simulink model "LQR_Kalman"  (R2024b)
settings: Solver=VariableStepAuto  StartTime=0.0  StopTime=tf  FixedStep=0.01  MaxStep=tf/1e4  RelTol=1e-4  AbsTol=1e-4
values from neighbouring files (symbols this model uses):
  A = [0 1; 0 0]    [Main_LQR_Kalman.m]    (also in dfdx.m = zeros(2))
  A_obs = A    [Main_LQR_Kalman.m]
  Bx = [0; Cx]    [Main_LQR_Kalman.m]
  Bx_obs = [Bx Kx_obs]    [Main_LQR_Kalman.m]
  By = [0; Cy]    [Main_LQR_Kalman.m]
  By_obs = [By Ky_obs]    [Main_LQR_Kalman.m]
  C = [1 0]    [Main_LQR_Kalman.m]
  C_obs = eye(2)    [Main_LQR_Kalman.m]
  D_obs = zeros(2)    [Main_LQR_Kalman.m]
  data_sys = [m r g J b lx ly]    [Main_LQR_Kalman.m]
  ICx_obs = [0 0]'    [Main_LQR_Kalman.m]
  ICy_obs = [0 0]'    [Main_LQR_Kalman.m]
  zx0 = [0.05,0]'    [Main_LQR_Kalman.m]
  zy0 = [0,0]'    [Main_LQR_Kalman.m]
settings Model: Creator=nicvi  LastModifiedBy=nicvi
settings SolverCC: AutoScaleAbsTol=off

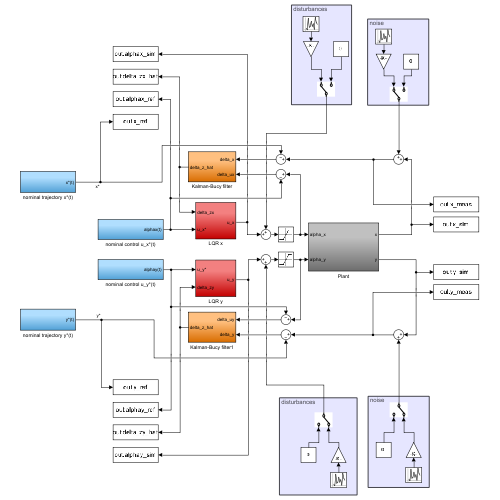
[thumbnail: Simulink's stored preview of the top-level diagram]
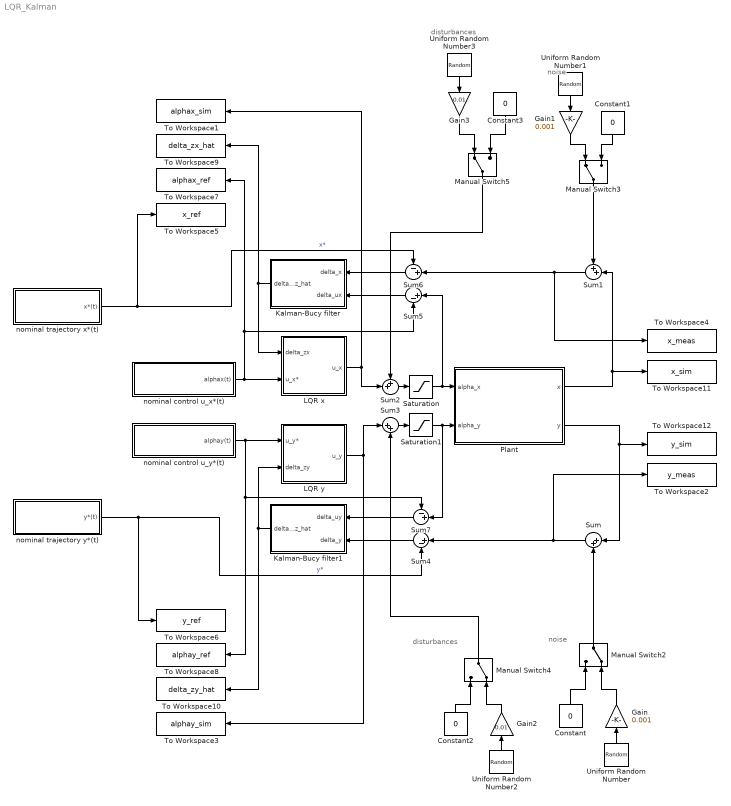
== system LQR_Kalman ==
  note: noise
  note: noise
  note: disturbances
  note: disturbances
  Constant{,1..3} (4 alike) : Constant  Value=0
  Gain : Gain  Gain=0.001
  Gain1 : Gain  Gain=0.001
  Gain2 : Gain  Gain=0.01
  Gain3 : Gain  Gain=0.01
  Kalman-Bucy filter : Subsystem
  Kalman-Bucy filter1 : Subsystem
  LQR x : Subsystem
  LQR y : Subsystem
  Manual Switch2 : ManualSwitch  CurrentSetting=0
  Manual Switch3 : ManualSwitch
  Manual Switch4 : ManualSwitch  CurrentSetting=0
  Manual Switch5 : ManualSwitch
  Plant : Subsystem
  Saturation : Saturate  UpperLimit=deg2rad(75)  LowerLimit=deg2rad(-75)
  Saturation1 : Saturate  UpperLimit=deg2rad(75)  LowerLimit=deg2rad(-75)
  Sum : Sum  Inputs=|++
  Sum1 : Sum  Inputs=++|
  Sum2 : Sum  Inputs=++|
  Sum3 : Sum  Inputs=|++
  Sum4 : Sum  Inputs=|+-
  Sum5 : Sum  Inputs=|+-
  Sum6 : Sum  Inputs=-+|
  Sum7 : Sum  Inputs=-+|
  To Workspace1 : ToWorkspace  VariableName=alphax_sim  SampleTime=-1
      settings: Save2DSignal=2-D array (concatenate along first dimension)
  To Workspace10 : ToWorkspace  VariableName=delta_zy_hat  SampleTime=-1
      settings: Save2DSignal=2-D array (concatenate along first dimension)
  To Workspace11 : ToWorkspace  VariableName=x_sim  SampleTime=-1
      settings: Save2DSignal=2-D array (concatenate along first dimension)
  To Workspace12 : ToWorkspace  VariableName=y_sim  SampleTime=-1
      settings: Save2DSignal=2-D array (concatenate along first dimension)
  To Workspace2 : ToWorkspace  VariableName=y_meas  SampleTime=-1
      settings: Save2DSignal=2-D array (concatenate along first dimension)
  To Workspace3 : ToWorkspace  VariableName=alphay_sim  SampleTime=-1
      settings: Save2DSignal=2-D array (concatenate along first dimension)
  To Workspace4 : ToWorkspace  VariableName=x_meas  SampleTime=-1
      settings: Save2DSignal=2-D array (concatenate along first dimension)
  To Workspace5 : ToWorkspace  VariableName=x_ref  SampleTime=-1
      settings: Save2DSignal=2-D array (concatenate along first dimension)
  To Workspace6 : ToWorkspace  VariableName=y_ref  SampleTime=-1
      settings: Save2DSignal=2-D array (concatenate along first dimension)
  To Workspace7 : ToWorkspace  VariableName=alphax_ref  SampleTime=-1
      settings: Save2DSignal=2-D array (concatenate along first dimension)
  To Workspace8 : ToWorkspace  VariableName=alphay_ref  SampleTime=-1
      settings: Save2DSignal=2-D array (concatenate along first dimension)
  To Workspace9 : ToWorkspace  VariableName=delta_zx_hat  SampleTime=-1
      settings: Save2DSignal=2-D array (concatenate along first dimension)
  Uniform Random Number : UniformRandomNumber  Minimum=-3  Maximum=3  SampleTime=0.01
  Uniform Random Number1 : UniformRandomNumber  Minimum=-3  Maximum=3  SampleTime=0.01
  Uniform Random Number2 : UniformRandomNumber  Minimum=-2  Maximum=2  SampleTime=0.01
  Uniform Random Number3 : UniformRandomNumber  Minimum=-2  Maximum=2  SampleTime=0.01
  nominal control u_x*(t) : Subsystem
  nominal control u_y*(t) : Subsystem
  nominal trajectory x*(t) : Subsystem
  nominal trajectory y*(t) : Subsystem
  wires:
  Manual Switch5/1 -> Sum2/1
  Uniform Random Number3/1 -> Gain3/1
  Gain2/1 -> Manual Switch4/2
  Constant2/1 -> Manual Switch4/1
  Gain1/1 -> Manual Switch3/1
  Plant/2(y) -> To Workspace12/1, Sum/1
  Sum7/1 -> Kalman-Bucy filter1/1(delta_uy)
  Uniform Random Number2/1 -> Gain2/1
  Gain/1 -> Manual Switch2/2
  nominal control u_y*(t)/1(alphay(t)) -> Sum7/1, To Workspace8/1, LQR y/1(u_y*)
  nominal control u_x*(t)/1(alphax(t)) -> Sum5/2, To Workspace7/1, LQR x/2(u_x*)
  Kalman-Bucy filter/1(delta_z_hat) -> To Workspace9/1, LQR x/1(delta_zx)
  LQR x/1(u_x) -> Sum2/2, To Workspace1/1
  Constant/1 -> Manual Switch2/1
  Sum6/1 -> Kalman-Bucy filter/1(delta_x)
  nominal trajectory x*(t)/1(x*(t)) -> Sum6/1, To Workspace5/1  "x*"
  Kalman-Bucy filter1/1(delta_z_hat) -> LQR y/2(delta_zy), To Workspace10/1
  Sum1/1 -> To Workspace4/1, Sum6/2
  Sum/1 -> To Workspace2/1, Sum4/1
  Saturation/1 -> Sum5/1, Plant/1(alpha_x)
  Uniform Random Number1/1 -> Gain1/1
  nominal trajectory y*(t)/1(y*(t)) -> Sum4/2, To Workspace6/1  "y*"
  Constant3/1 -> Manual Switch5/2
  Manual Switch2/1 -> Sum/2
  Manual Switch3/1 -> Sum1/1
  Sum4/1 -> Kalman-Bucy filter1/2(delta_y)
  Gain3/1 -> Manual Switch5/1
  Sum5/1 -> Kalman-Bucy filter/2(delta_ux)
  Uniform Random Number/1 -> Gain/1
  Manual Switch4/1 -> Sum3/2
  Plant/1(x) -> To Workspace11/1, Sum1/2
  Constant1/1 -> Manual Switch3/2
  Sum2/1 -> Saturation/1
  Sum3/1 -> Saturation1/1
  LQR y/1(u_y) -> Sum3/1, To Workspace3/1
  Saturation1/1 -> Sum7/2, Plant/2(alpha_y)

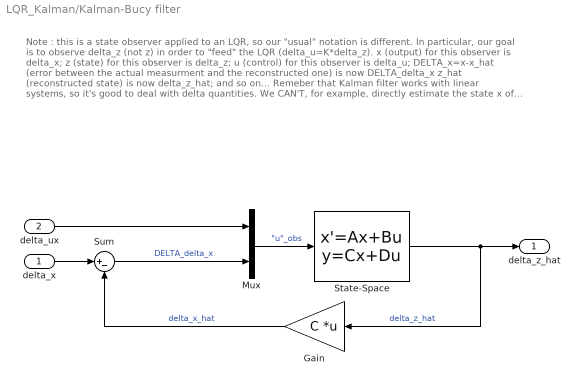
== system LQR_Kalman/Kalman-Bucy filter ==
  note: Note : this is a state observer applied to an LQR, so our "usual" notation is different. In particular, our goal is to observe delta_z (not z) in order to "feed" the LQR (delta_u=K*delta_z).
      |
      | x (output) for this observer is delta_x;
      | z (state) for this observer is delta_z;
      | u (control) for this observer is delta_u;
      | DELTA_x=x-x_hat (error between the actual measurment and the reconstructed one) is now DELTA_delta_x
      | z_hat (reconstructed state) is now delta_z_hat;
      | and so on...
      |
      | Remeber that Kalman filter works with linear systems, so it's good to deal with delta quantities. We CAN'T, for example, directly estimate the state x of the nonlinear system (we need a nonlinear observer for that, for exemple an extension of Kalman filter).
  delta_x : Inport
  delta_ux : Inport  Port=2
  Gain : Gain  Gain=C  Multiplication=Matrix(K*u) (u vector)
  Mux : Mux  Inputs=2
  State-Space : StateSpace  A=A_obs  B=Bx_obs  C=C_obs  D=D_obs  InitialCondition=ICx_obs
  Sum : Sum  Inputs=|+-
  delta_z_hat : Outport
  wires:
  Gain/1 -> Sum/2  "delta_x_hat"
  delta_x/1 -> Sum/1
  Sum/1 -> Mux/2  "DELTA_delta_x"
  Mux/1 -> State-Space/1  "\"u\"_obs"
  delta_ux/1 -> Mux/1
  State-Space/1 -> Gain/1, delta_z_hat/1  "delta_z_hat"

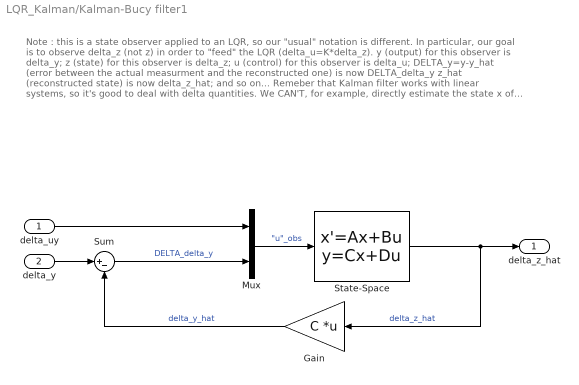
== system LQR_Kalman/Kalman-Bucy filter1 ==
  note: Note : this is a state observer applied to an LQR, so our "usual" notation is different. In particular, our goal is to observe delta_z (not z) in order to "feed" the LQR (delta_u=K*delta_z).
      |
      | y (output) for this observer is delta_y;
      | z (state) for this observer is delta_z;
      | u (control) for this observer is delta_u;
      | DELTA_y=y-y_hat (error between the actual measurment and the reconstructed one) is now DELTA_delta_y
      | z_hat (reconstructed state) is now delta_z_hat;
      | and so on...
      |
      | Remeber that Kalman filter works with linear systems, so it's good to deal with delta quantities. We CAN'T, for example, directly estimate the state x of the nonlinear system (we need a nonlinear observer for that, for exemple an extension of Kalman filter).
  delta_uy : Inport
  delta_y : Inport  Port=2
  Gain : Gain  Gain=C  Multiplication=Matrix(K*u) (u vector)
  Mux : Mux  Inputs=2
  State-Space : StateSpace  A=A_obs  B=By_obs  C=C_obs  D=D_obs  InitialCondition=ICy_obs
  Sum : Sum  Inputs=|+-
  delta_z_hat : Outport
  wires:
  State-Space/1 -> delta_z_hat/1, Gain/1  "delta_z_hat"
  delta_uy/1 -> Mux/1
  Mux/1 -> State-Space/1  "\"u\"_obs"
  Sum/1 -> Mux/2  "DELTA_delta_y"
  delta_y/1 -> Sum/1
  Gain/1 -> Sum/2  "delta_y_hat"

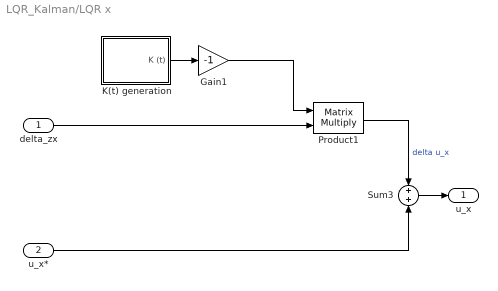
== system LQR_Kalman/LQR x ==
  delta_zx : Inport
  u_x* : Inport  Port=2
  Gain1 : Gain  Gain=-1
  K(t) generation : Subsystem
  Product1 : Product  Multiplication=Matrix(*)
  Sum3 : Sum
  u_x : Outport
  wires:
  delta_zx/1 -> Product1/2
  Product1/1 -> Sum3/1  "delta u_x"
  K(t) generation/1(K (t)) -> Gain1/1
  Gain1/1 -> Product1/1
  Sum3/1 -> u_x/1
  u_x*/1 -> Sum3/2

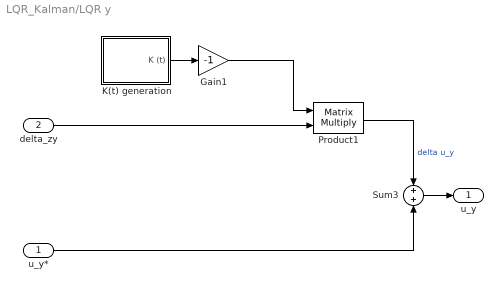
== system LQR_Kalman/LQR y ==
  u_y* : Inport
  delta_zy : Inport  Port=2
  Gain1 : Gain  Gain=-1
  K(t) generation : Subsystem
  Product1 : Product  Multiplication=Matrix(*)
  Sum3 : Sum
  u_y : Outport
  wires:
  u_y*/1 -> Sum3/2
  Sum3/1 -> u_y/1
  Gain1/1 -> Product1/1
  K(t) generation/1(K (t)) -> Gain1/1
  Product1/1 -> Sum3/1  "delta u_y"
  delta_zy/1 -> Product1/2

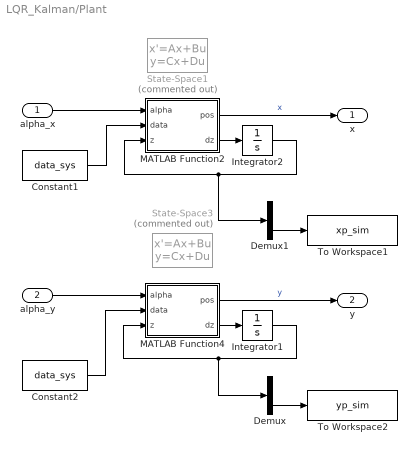
== system LQR_Kalman/Plant ==
  alpha_x : Inport
  alpha_y : Inport  Port=2
  Constant1 : Constant  Value=data_sys
  Constant2 : Constant  Value=data_sys
  Demux : Demux  Outputs=2
  Demux1 : Demux  Outputs=2
  Integrator1 : Integrator  InitialCondition=zy0
  Integrator2 : Integrator  InitialCondition=zx0
  MATLAB Function2 : MATLAB Function  TreatAsAtomicUnit=on
  MATLAB Function4 : MATLAB Function  TreatAsAtomicUnit=on
  State-Space1 : StateSpace  Commented=on  A=A  B=Bx  C=C  D=0  InitialCondition=zx0
  State-Space3 : StateSpace  Commented=on  A=A  B=By  C=C  D=0  InitialCondition=zy0
  To Workspace1 : ToWorkspace  VariableName=xp_sim  SampleTime=-1
      settings: Save2DSignal=2-D array (concatenate along first dimension)
  To Workspace2 : ToWorkspace  VariableName=yp_sim  SampleTime=-1
      settings: Save2DSignal=2-D array (concatenate along first dimension)
  x : Outport
  y : Outport  Port=2
  wires:
  alpha_y/1 -> MATLAB Function4/1(alpha)
  alpha_x/1 -> MATLAB Function2/1(alpha)
  MATLAB Function2/1(pos) -> x/1  "x"
  Constant1/1 -> MATLAB Function2/2(data)
  MATLAB Function2/2(dz) -> Integrator2/1
  Integrator2/1 -> Demux1/1, MATLAB Function2/3(z)
  MATLAB Function4/2(dz) -> Integrator1/1
  Integrator1/1 -> Demux/1, MATLAB Function4/3(z)
  Constant2/1 -> MATLAB Function4/2(data)
  MATLAB Function4/1(pos) -> y/1  "y"
  Demux/2 -> To Workspace2/1
  Demux1/2 -> To Workspace1/1

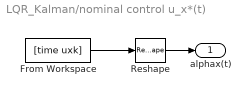
== system LQR_Kalman/nominal control u_x*(t) ==
  From Workspace : FromWorkspace  VariableName=[time uxk]
  Reshape : Reshape  OutputDimensionality=Column vector (2-D)
  alphax(t) : Outport
  wires:
  From Workspace/1 -> Reshape/1
  Reshape/1 -> alphax(t)/1

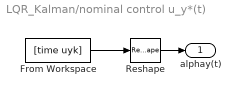
== system LQR_Kalman/nominal control u_y*(t) ==
  From Workspace : FromWorkspace  VariableName=[time uyk]
  Reshape : Reshape  OutputDimensionality=Column vector (2-D)
  alphay(t) : Outport
  wires:
  From Workspace/1 -> Reshape/1
  Reshape/1 -> alphay(t)/1

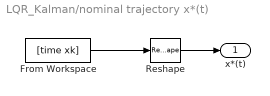
== system LQR_Kalman/nominal trajectory x*(t) ==
  From Workspace : FromWorkspace  VariableName=[time xk]
  Reshape : Reshape  OutputDimensionality=Column vector (2-D)
  x*(t) : Outport
  wires:
  From Workspace/1 -> Reshape/1
  Reshape/1 -> x*(t)/1

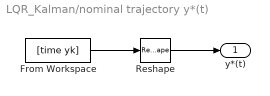
== system LQR_Kalman/nominal trajectory y*(t) ==
  From Workspace : FromWorkspace  VariableName=[time yk]
  Reshape : Reshape  OutputDimensionality=Column vector (2-D)
  y*(t) : Outport
  wires:
  From Workspace/1 -> Reshape/1
  Reshape/1 -> y*(t)/1

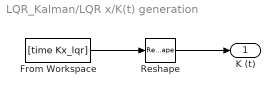
== system LQR_Kalman/LQR x/K(t) generation ==
  From Workspace : FromWorkspace  VariableName=[time Kx_lqr]
  Reshape : Reshape  OutputDimensionality=Row vector (2-D)
  K (t) : Outport
  wires:
  Reshape/1 -> K (t)/1
  From Workspace/1 -> Reshape/1

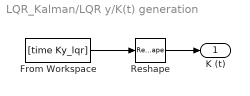
== system LQR_Kalman/LQR y/K(t) generation ==
  From Workspace : FromWorkspace  VariableName=[time Ky_lqr]
  Reshape : Reshape  OutputDimensionality=Row vector (2-D)
  K (t) : Outport
  wires:
  From Workspace/1 -> Reshape/1
  Reshape/1 -> K (t)/1

== matlab function LQR_Kalman/Plant/MATLAB Function4 ==
  data: pos output; alpha input; dz output; data input; z input
function [pos,dz] = fcn(alpha,data,z)

m=data(1);
r=data(2);
g=data(3);
J=data(4);
b=data(5);
ly=data(7);

Cx=m*g*b/(m+J/r^2)/ly;

dz=zeros(2,1);
dz(1)=z(2);
dz(2)=Cx*sin(alpha);

pos=z(1);

end

== matlab function LQR_Kalman/Plant/MATLAB Function2 ==
  data: pos output; alpha input; dz output; data input; z input
function [pos,dz] = fcn(alpha,data,z)

m=data(1);
r=data(2);
g=data(3);
J=data(4);
b=data(5);
lx=data(6);

Cx=m*g*b/(m+J/r^2)/lx;

dz=zeros(2,1);
dz(1)=z(2);
dz(2)=Cx*sin(alpha);

pos=z(1);

end
